simulink model "OpenEndWinding_withDirect_Control"  (R2023b)
settings: Solver=VariableStepAuto  StartTime=0.0  StopTime=0.2  RelTol=1e-3  AbsTol=1e-3  EnableMultiTasking=on
values from neighbouring files (symbols this model uses):
  Amplitude = 0.9    [OpenEndWinding_sim.m]
  elec_freq = 5000/60* 4    (= 333.333333333)    [OpenEndWinding_sim.m]
  FSW = 36000    [OpenEndWinding_sim.m]
  Ki = C.Ki    [OpenEndWinding_sim.m]
  Kp = C.Kp    [OpenEndWinding_sim.m]
  Psi1_f = 0.05    [OpenEndWinding_sim.m]
  Rm = 10e-3    (= 0.01)    [OpenEndWinding_sim.m]
  sample_time = 1e-6    (= 1e-06)    [OpenEndWinding_sim.m]
libraries: nesl_utility x29, ee_lib x27, fl_lib x16, eeGeneralControl x5, spsRMSLib x5, spsTriangleGeneratorLib x2, simulink x2, eeLCFB1 x1, slpidlib x1, spsabctodq0Lib x1, spspowerguiLib x1
(part 2 of 2)

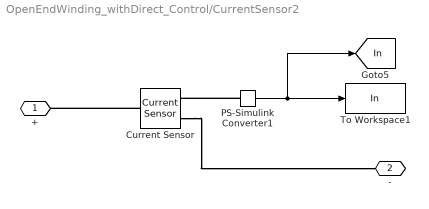
== system OpenEndWinding_withDirect_Control/CurrentSensor2 ==
  Current Sensor : fl_lib/Electrical/Electrical Sensors/Current Sensor
  PS-Simulink Converter1 : nesl_utility/PS-Simulink Converter  PhysicalDomain=network_engine_domain  SubClassName=ps_output  LeftPortType=input  RightPortType=output  PseudoPeriodic=off  Frequencies=[]  VectorFormat=1-D array  Unit=A  AffineConversion=off
  To Workspace1 : ToWorkspace  VariableName=In  SampleTime=SampleTime
  + : PMIOPort  Side=Left
  - : PMIOPort  Port=2  Side=Right
  tag scope: In=global
  wires:
  PS-Simulink Converter1/1 -> [In], To Workspace1/1
  connections:
  Current Sensor/RConn2 -- -/RConn1
  Current Sensor/LConn1 -- +/RConn1
  PS-Simulink Converter1/LConn1 -- Current Sensor/RConn1

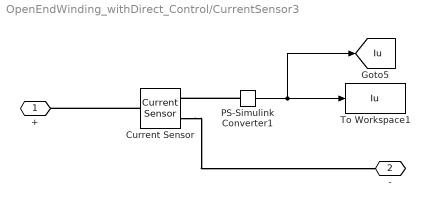
== system OpenEndWinding_withDirect_Control/CurrentSensor3 ==
  Current Sensor : fl_lib/Electrical/Electrical Sensors/Current Sensor
  PS-Simulink Converter1 : nesl_utility/PS-Simulink Converter  PhysicalDomain=network_engine_domain  SubClassName=ps_output  LeftPortType=input  RightPortType=output  PseudoPeriodic=off  Frequencies=[]  VectorFormat=1-D array  Unit=A  AffineConversion=off
  To Workspace1 : ToWorkspace  VariableName=Iu  SampleTime=SampleTime
  + : PMIOPort  Side=Left
  - : PMIOPort  Port=2  Side=Right
  tag scope: Iu=global
  wires:
  PS-Simulink Converter1/1 -> [Iu], To Workspace1/1
  connections:
  Current Sensor/RConn2 -- -/RConn1
  Current Sensor/LConn1 -- +/RConn1
  PS-Simulink Converter1/LConn1 -- Current Sensor/RConn1

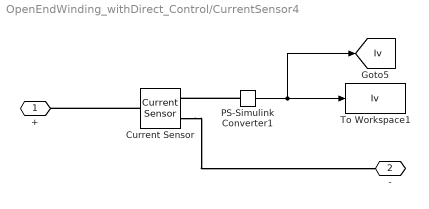
== system OpenEndWinding_withDirect_Control/CurrentSensor4 ==
  Current Sensor : fl_lib/Electrical/Electrical Sensors/Current Sensor
  PS-Simulink Converter1 : nesl_utility/PS-Simulink Converter  PhysicalDomain=network_engine_domain  SubClassName=ps_output  LeftPortType=input  RightPortType=output  PseudoPeriodic=off  Frequencies=[]  VectorFormat=1-D array  Unit=A  AffineConversion=off
  To Workspace1 : ToWorkspace  VariableName=Iv  SampleTime=SampleTime
  + : PMIOPort  Side=Left
  - : PMIOPort  Port=2  Side=Right
  tag scope: Iv=global
  wires:
  PS-Simulink Converter1/1 -> [Iv], To Workspace1/1
  connections:
  Current Sensor/RConn2 -- -/RConn1
  Current Sensor/LConn1 -- +/RConn1
  PS-Simulink Converter1/LConn1 -- Current Sensor/RConn1

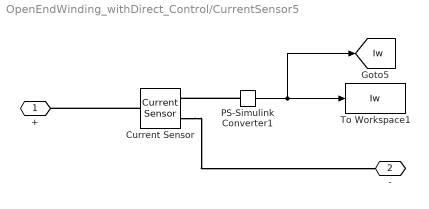
== system OpenEndWinding_withDirect_Control/CurrentSensor5 ==
  Current Sensor : fl_lib/Electrical/Electrical Sensors/Current Sensor
  PS-Simulink Converter1 : nesl_utility/PS-Simulink Converter  PhysicalDomain=network_engine_domain  SubClassName=ps_output  LeftPortType=input  RightPortType=output  PseudoPeriodic=off  Frequencies=[]  VectorFormat=1-D array  Unit=A  AffineConversion=off
  To Workspace1 : ToWorkspace  VariableName=Iw  SampleTime=SampleTime
  + : PMIOPort  Side=Left
  - : PMIOPort  Port=2  Side=Right
  tag scope: Iw=global
  wires:
  PS-Simulink Converter1/1 -> [Iw], To Workspace1/1
  connections:
  Current Sensor/RConn2 -- -/RConn1
  Current Sensor/LConn1 -- +/RConn1
  PS-Simulink Converter1/LConn1 -- Current Sensor/RConn1

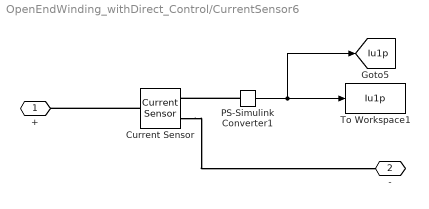
== system OpenEndWinding_withDirect_Control/CurrentSensor6 ==
  Current Sensor : fl_lib/Electrical/Electrical Sensors/Current Sensor
  PS-Simulink Converter1 : nesl_utility/PS-Simulink Converter  PhysicalDomain=network_engine_domain  SubClassName=ps_output  LeftPortType=input  RightPortType=output  PseudoPeriodic=off  Frequencies=[]  VectorFormat=1-D array  Unit=A  AffineConversion=off
  To Workspace1 : ToWorkspace  VariableName=Iu1p  SampleTime=SampleTime
  + : PMIOPort  Side=Left
  - : PMIOPort  Port=2  Side=Right
  tag scope: Iu1p=global
  wires:
  PS-Simulink Converter1/1 -> [Iu1p], To Workspace1/1
  connections:
  Current Sensor/RConn2 -- -/RConn1
  Current Sensor/LConn1 -- +/RConn1
  PS-Simulink Converter1/LConn1 -- Current Sensor/RConn1

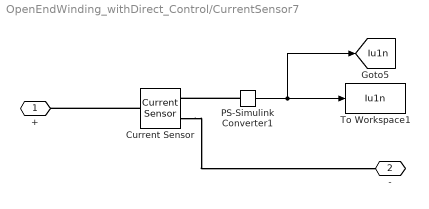
== system OpenEndWinding_withDirect_Control/CurrentSensor7 ==
  Current Sensor : fl_lib/Electrical/Electrical Sensors/Current Sensor
  PS-Simulink Converter1 : nesl_utility/PS-Simulink Converter  PhysicalDomain=network_engine_domain  SubClassName=ps_output  LeftPortType=input  RightPortType=output  PseudoPeriodic=off  Frequencies=[]  VectorFormat=1-D array  Unit=A  AffineConversion=off
  To Workspace1 : ToWorkspace  VariableName=Iu1n  SampleTime=SampleTime
  + : PMIOPort  Side=Left
  - : PMIOPort  Port=2  Side=Right
  tag scope: Iu1n=global
  wires:
  PS-Simulink Converter1/1 -> [Iu1n], To Workspace1/1
  connections:
  Current Sensor/RConn2 -- -/RConn1
  Current Sensor/LConn1 -- +/RConn1
  PS-Simulink Converter1/LConn1 -- Current Sensor/RConn1

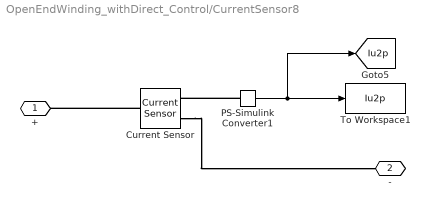
== system OpenEndWinding_withDirect_Control/CurrentSensor8 ==
  Current Sensor : fl_lib/Electrical/Electrical Sensors/Current Sensor
  PS-Simulink Converter1 : nesl_utility/PS-Simulink Converter  PhysicalDomain=network_engine_domain  SubClassName=ps_output  LeftPortType=input  RightPortType=output  PseudoPeriodic=off  Frequencies=[]  VectorFormat=1-D array  Unit=A  AffineConversion=off
  To Workspace1 : ToWorkspace  VariableName=Iu2p  SampleTime=SampleTime
  + : PMIOPort  Side=Left
  - : PMIOPort  Port=2  Side=Right
  tag scope: Iu2p=global
  wires:
  PS-Simulink Converter1/1 -> [Iu2p], To Workspace1/1
  connections:
  Current Sensor/RConn2 -- -/RConn1
  Current Sensor/LConn1 -- +/RConn1
  PS-Simulink Converter1/LConn1 -- Current Sensor/RConn1

== system OpenEndWinding_withDirect_Control/CurrentSensor9 ==
  Current Sensor : fl_lib/Electrical/Electrical Sensors/Current Sensor
  PS-Simulink Converter1 : nesl_utility/PS-Simulink Converter  PhysicalDomain=network_engine_domain  SubClassName=ps_output  LeftPortType=input  RightPortType=output  PseudoPeriodic=off  Frequencies=[]  VectorFormat=1-D array  Unit=A  AffineConversion=off
  To Workspace1 : ToWorkspace  VariableName=Iu2n  SampleTime=SampleTime
  + : PMIOPort  Side=Left
  - : PMIOPort  Port=2  Side=Right
  tag scope: Iu2n=global
  wires:
  PS-Simulink Converter1/1 -> [Iu2n], To Workspace1/1
  connections:
  Current Sensor/RConn2 -- -/RConn1
  Current Sensor/LConn1 -- +/RConn1
  PS-Simulink Converter1/LConn1 -- Current Sensor/RConn1

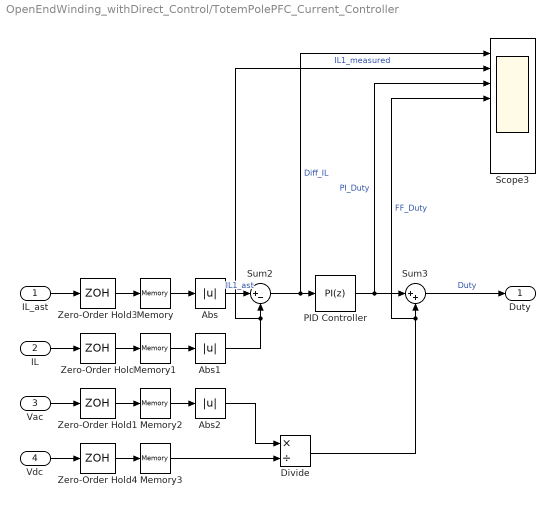
== system OpenEndWinding_withDirect_Control/TotemPolePFC_Current_Controller ==
  IL_ast : Inport
  IL : Inport  Port=2
  Vac : Inport  Port=3
  Vdc : Inport  Port=4
  Abs : Abs  SaturateOnIntegerOverflow=off
  Abs1 : Abs  SaturateOnIntegerOverflow=off
  Abs2 : Abs  SaturateOnIntegerOverflow=off
  Divide : Product  Inputs=*/
  Memory{,1..3} (4 alike) : Memory
  PID Controller : slpidlib/PID Controller  Controller=PI  Form=Parallel  TimeDomain=Discrete-time  UseExternalTs=off  SampleTime=1/FSW  IntegratorMethod=Forward Euler  FilterMethod=Forward Euler  ControllerParametersSource=internal  P=Kp  I=Ki  UseKiTs=off  D=0  N=100  UseFilter=on  TunerSelectOption=Transfer Function Based (PID Tuner App)  InitialConditionSource=internal  InitialConditionForIntegrator=0  InitialConditionForFilter=0  DifferentiatorICPrevScaledInput=0  ExternalReset=none  TrackingMode=off  Kt=1  LimitOutput=on  SatLimitsSource=internal  UpperSaturationLimit=0.95  LowerSaturationLimit=0  LinearizeAsGain=on  AntiWindupMode=clamping  Kb=1  LimitIntegrator=off  UpperIntegratorSaturationLimit=inf  LowerIntegratorSaturationLimit=-inf  POutMin=[]  POutMax=[]  IOutMin=[]  IOutMax=[]  DOutMin=[]  DOutMax=[]  NOutMin=[]  NOutMax=[]  SumOutMin=[]  SumOutMax=[]  SaturationOutMin=[]  SaturationOutMax=[]  PParamMin=[]  PParamMax=[]  IParamMin=[]  IParamMax=[]  DParamMin=[]  DParamMax=[]  NParamMin=[]  NParamMax=[]  KbParamMin=[]  KbParamMax=[]  KtParamMin=[]  KtParamMax=[]  KbOutMin=[]  KbOutMax=[]  KtOutMin=[]  KtOutMax=[]  IntegratorOutMin=[]  IntegratorOutMax=[]  FilterOutMin=[]  FilterOutMax=[]  SumI1OutMin=[]  SumI1OutMax=[]  SumI2OutMin=[]  SumI2OutMax=[]  SumI3OutMin=[]  SumI3OutMax=[]  SumI4OutMin=[]  SumI4OutMax=[]  SumDOutMin=[]  SumDOutMax=[]  DifferentiatorOutMin=[]  DifferentiatorOutMax=[]  FilterDiffOutCoefMin=[]  FilterDiffOutCoefMax=[]  ReciprocalOutMin=[]  ReciprocalOutMax=[]  SumDenOutMin=[]  SumDenOutMax=[]  SumNumOutMin=[]  SumNumOutMax=[]  DivideOutMin=[]  DivideOutMax=[]  UdiffTsProdOutMin=[]  UdiffTsProdOutMax=[]  NTsProdOutMin=[]  NTsProdOutMax=[]  UintegralTsProdOutMin=[]  UintegralTsProdOutMax=[]  UngainTsProdOutMin=[]  UngainTsProdOutMax=[]  ClampingZeroOutDataTypeStr=Inherit: Inherit via back propagation  ClampingZeroOutMin=[]  ClampingZeroOutMax=[]  FilterDenConstantOutDataTypeStr=Inherit: Inherit via back propagation  FilterDenConstantOutMin=[]  FilterDenConstantOutMax=[]  PCopyOutDataTypeStr=Inherit: Inherit via back propagation  PCopyOutMin=[]  PCopyOutMax=[]  NCopyOutDataTypeStr=Inherit: Inherit via back propagation  NCopyOutMin=[]  NCopyOutMax=[]  IntegratorContinuousStateAttributes=''  IntegratorStateMustResolveToSignalObject=off  IntegratorRTWStateStorageClass=Auto  FilterContinuousStateAttributes=''  FilterStateMustResolveToSignalObject=off  FilterRTWStateStorageClass=Auto  ParallelPVariant=InternalParameters  IdealPVariant=Disabled  IVariant=InternalParameters  DVariant=Disabled  IntegratorVariant=Discrete  SatVariant=Enabled  AWVariant=DiscClampingParallel  PCopyVariant=Disabled  TRVariant=Disabled  FdbkBlocksVariant=Forward  IdealPFdbkVariant=Disabled  SatFdbkVariant=Disabled  DerivativeFilterVariant=Disabled  NVariant=Disabled  NCopyVariant=Disabled_SignalSpec  FilterICVariant=Disabled  IntegratorICVariant=InternalICs  ExternalResetVariant=Disabled  TRSumVariant=Passthrough  SumFdbkVariant=Disabled  SumVariant=Sum_PI  TsampFilterVariant=InternalTs  TsampNgainVariant=Passthrough  TsampIntegralVariant=Disabled_SignalSpec  ExternalSaturationOutDataTypeStr=Inherit: Same as second input
  Scope3 : Scope  NumInputPorts=8
  Sum2 : Sum  Inputs=|+-
  Sum3 : Sum  Inputs=|++
  Zero-Order Hold{,1,3..4} (4 alike) : ZeroOrderHold  SampleTime=1/FSW
  Duty : Outport
  wires:
  Zero-Order Hold3/1 -> Memory/1
  Memory1/1 -> Abs1/1
  PID Controller/1 -> Scope3/3, Sum3/1  "PI_Duty"
  Abs1/1 -> Scope3/2, Sum2/2  "IL1_measured"
  Zero-Order Hold/1 -> Memory1/1
  Divide/1 -> Scope3/4, Sum3/2  "FF_Duty"
  Zero-Order Hold1/1 -> Memory2/1
  Zero-Order Hold4/1 -> Memory3/1
  Sum3/1 -> Duty/1  "Duty"
  Sum2/1 -> Scope3/1, PID Controller/1  "Diff_IL"
  Memory2/1 -> Abs2/1
  Vdc/1 -> Zero-Order Hold4/1
  Vac/1 -> Zero-Order Hold1/1
  Memory/1 -> Abs/1
  Abs/1 -> Sum2/1  "IL1_ast"
  Abs2/1 -> Divide/1
  Memory3/1 -> Divide/2
  IL_ast/1 -> Zero-Order Hold3/1
  IL/1 -> Zero-Order Hold/1

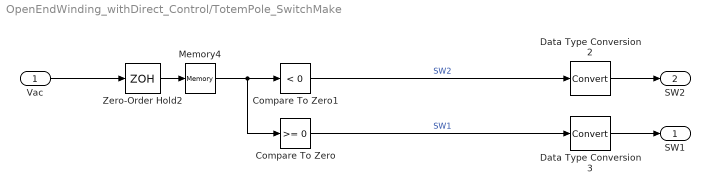
== system OpenEndWinding_withDirect_Control/TotemPole_SwitchMake ==
  Vac : Inport
  Compare To Zero : simulink/Logic and Bit Operations/Compare To Zero  relop=>=  OutDataTypeStr=boolean
  Compare To Zero1 : simulink/Logic and Bit Operations/Compare To Zero  relop=<  OutDataTypeStr=boolean
  Data Type Conversion2 : DataTypeConversion  SaturateOnIntegerOverflow=off  RndMeth=Floor
  Data Type Conversion3 : DataTypeConversion  SaturateOnIntegerOverflow=off  RndMeth=Floor
  Memory4 : Memory
  Zero-Order Hold2 : ZeroOrderHold  SampleTime=1/FSW
  SW1 : Outport
  SW2 : Outport  Port=2
  wires:
  Compare To Zero/1 -> Data Type Conversion3/1  "SW1"
  Memory4/1 -> Compare To Zero/1, Compare To Zero1/1
  Vac/1 -> Zero-Order Hold2/1
  Zero-Order Hold2/1 -> Memory4/1
  Compare To Zero1/1 -> Data Type Conversion2/1  "SW2"
  Data Type Conversion3/1 -> SW1/1
  Data Type Conversion2/1 -> SW2/1

== system OpenEndWinding_withDirect_Control/VoltageSensor ==
  PS-Simulink Converter1 : nesl_utility/PS-Simulink Converter  PhysicalDomain=network_engine_domain  SubClassName=ps_output  LeftPortType=input  RightPortType=output  PseudoPeriodic=off  Frequencies=[]  VectorFormat=1-D array  Unit=V  AffineConversion=off
  To Workspace1 : ToWorkspace  VariableName=Vin  SampleTime=SampleTime
  Voltage Sensor : fl_lib/Electrical/Electrical Sensors/Voltage Sensor
  + : PMIOPort  Side=Left
  - : PMIOPort  Port=2  Side=Left
  tag scope: Vin=global
  wires:
  PS-Simulink Converter1/1 -> To Workspace1/1, [Vin]
  connections:
  Voltage Sensor/RConn1 -- PS-Simulink Converter1/LConn1
  Voltage Sensor/RConn2 -- -/RConn1
  Voltage Sensor/LConn1 -- +/RConn1

== system OpenEndWinding_withDirect_Control/VoltageSensor1 ==
  PS-Simulink Converter1 : nesl_utility/PS-Simulink Converter  PhysicalDomain=network_engine_domain  SubClassName=ps_output  LeftPortType=input  RightPortType=output  PseudoPeriodic=off  Frequencies=[]  VectorFormat=1-D array  Unit=V  AffineConversion=off
  To Workspace1 : ToWorkspace  VariableName=Vu1_n  SampleTime=SampleTime
  Voltage Sensor : fl_lib/Electrical/Electrical Sensors/Voltage Sensor
  + : PMIOPort  Side=Left
  - : PMIOPort  Port=2  Side=Left
  tag scope: Vu1_n=global
  wires:
  PS-Simulink Converter1/1 -> To Workspace1/1, [Vu1_n]
  connections:
  Voltage Sensor/RConn1 -- PS-Simulink Converter1/LConn1
  Voltage Sensor/RConn2 -- -/RConn1
  Voltage Sensor/LConn1 -- +/RConn1

== system OpenEndWinding_withDirect_Control/Vu ==
  PS-Simulink Converter1 : nesl_utility/PS-Simulink Converter  PhysicalDomain=network_engine_domain  SubClassName=ps_output  LeftPortType=input  RightPortType=output  PseudoPeriodic=off  Frequencies=[]  VectorFormat=1-D array  Unit=V  AffineConversion=off
  To Workspace1 : ToWorkspace  VariableName=Vu  SampleTime=SampleTime
  Voltage Sensor : fl_lib/Electrical/Electrical Sensors/Voltage Sensor
  + : PMIOPort  Side=Left
  - : PMIOPort  Port=2  Side=Left
  tag scope: Vu=global
  wires:
  PS-Simulink Converter1/1 -> To Workspace1/1, [Vu]
  connections:
  Voltage Sensor/RConn1 -- PS-Simulink Converter1/LConn1
  Voltage Sensor/RConn2 -- -/RConn1
  Voltage Sensor/LConn1 -- +/RConn1

== system OpenEndWinding_withDirect_Control/Vv ==
  PS-Simulink Converter1 : nesl_utility/PS-Simulink Converter  PhysicalDomain=network_engine_domain  SubClassName=ps_output  LeftPortType=input  RightPortType=output  PseudoPeriodic=off  Frequencies=[]  VectorFormat=1-D array  Unit=V  AffineConversion=off
  To Workspace1 : ToWorkspace  VariableName=Vv  SampleTime=SampleTime
  Voltage Sensor : fl_lib/Electrical/Electrical Sensors/Voltage Sensor
  + : PMIOPort  Side=Left
  - : PMIOPort  Port=2  Side=Left
  tag scope: Vv=global
  wires:
  PS-Simulink Converter1/1 -> To Workspace1/1, [Vv]
  connections:
  Voltage Sensor/RConn1 -- PS-Simulink Converter1/LConn1
  Voltage Sensor/RConn2 -- -/RConn1
  Voltage Sensor/LConn1 -- +/RConn1

== system OpenEndWinding_withDirect_Control/Vw ==
  PS-Simulink Converter1 : nesl_utility/PS-Simulink Converter  PhysicalDomain=network_engine_domain  SubClassName=ps_output  LeftPortType=input  RightPortType=output  PseudoPeriodic=off  Frequencies=[]  VectorFormat=1-D array  Unit=V  AffineConversion=off
  To Workspace1 : ToWorkspace  VariableName=Vw  SampleTime=SampleTime
  Voltage Sensor : fl_lib/Electrical/Electrical Sensors/Voltage Sensor
  + : PMIOPort  Side=Left
  - : PMIOPort  Port=2  Side=Left
  tag scope: Vw=global
  wires:
  PS-Simulink Converter1/1 -> To Workspace1/1, [Vw]
  connections:
  Voltage Sensor/RConn1 -- PS-Simulink Converter1/LConn1
  Voltage Sensor/RConn2 -- -/RConn1
  Voltage Sensor/LConn1 -- +/RConn1
